simulink model "IsolatedUDP_v2"  (R2020a)
settings: Solver=FixedStepAuto  StartTime=0.0  StopTime=inf  FixedStep=0.001  RelTol=1e-3  EnableMultiTasking=on
undefined symbols (not defined in the file): daq
libraries: instrumentlib x2, dspstat3 x2, dspsigops x2, daqlib x1, quarc_library x1
settings Model: SimulationMode=accelerator  ExtModeTrigDuration=10000  Creator=pthms  LastModifiedBy=jacksonbremen
settings SolverCC: ConcurrentTasks=on  PositivePriorityOrder=on  AutoInsertRateTranBlk=on  InsertRTBMode=Never (minimum delay)
settings DataIOCC: ReturnWorkspaceOutputs=off
settings DebuggingCC: ArithmeticOperatorsInVariantConditions=warning
settings SFSimCC: SimUseLocalCustomCode=off  CustomCodeUndefinedFunction=UseInterfaceOnly
settings RTWCC: Description=QUARC Win64 Target  SystemTargetFile=quarc_win64.tlc  TemplateMakefile=quarc_default_tmf  RTWUseLocalCustomCode=off
settings STFCustomTargetCC: TargetPreCompLibLocation=C:\PROGRA~3\QUARC\lib\2018a\win64\release  TargetLangStandard=C99 (ISO)  ConcurrentExecutionCompliant=on  GRTInterface=on  SystemTargetFile=quarc_win64.tlc
settings GRTTargetCC: TargetPreCompLibLocation=C:\PROGRA~3\QUARC\lib\2018a\win64\release  ParMdlRefBuildCompliant=off  CompOptLevelCompliant=off  CombineOutputUpdateFcns=off  MatFileLogging=off  CPPClassGenCompliant=off  GRTInterface=on  UseToolchainInfoCompliant=off  ExtMode=on  ExtModeMexFile=quarc_comm

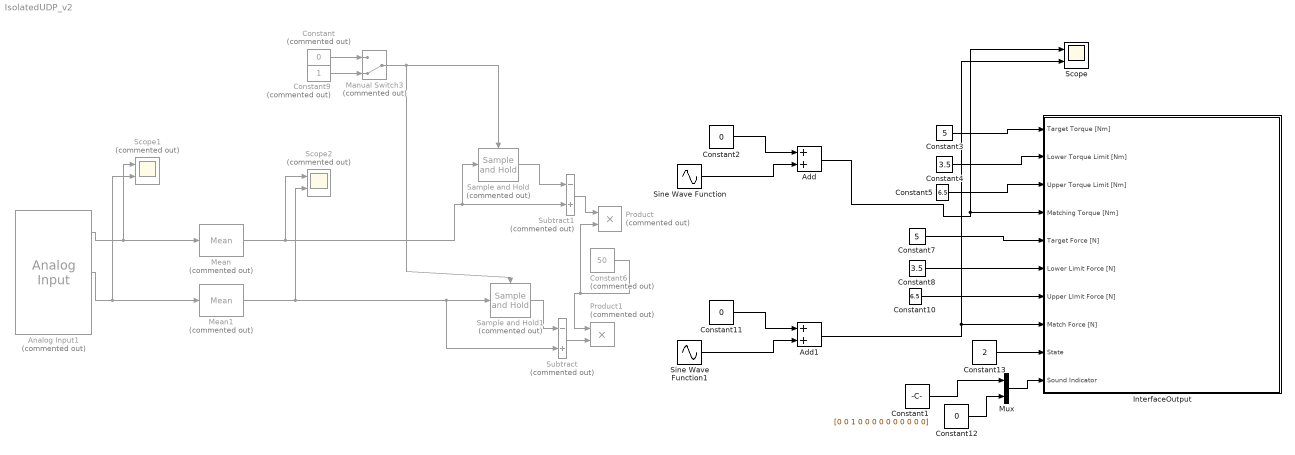
== system IsolatedUDP_v2 ==
  Add : Sum
  Add1 : Sum
  Analog Input1 : daqlib/Analog Input  Commented=on  DeviceMenu=ni Dev1 (USB-6229 (OEM))  Device=ni Dev1 (USB-6229 (OEM))  ObjConstructor=daq.createSession('ni')  NChannelsSelected=2  Channels=1$ai0$$Dev1$1$4$3$1$#1$ai1$$Dev1$1$4$3$1$#0$ai2$$Dev1$1$4$3$1$#0$ai3$$Dev1$1$4$3$1$#0$ai4$$Dev1$1$4$3$1$#0$ai5$$Dev1$1$4$3$1$#0$ai6$$Dev1$1$4$3$1$#0$ai7$$Dev1$1$4$3$1$#0$ai8$$Dev1$1$4$1$1$#0$ai9$$Dev1$1$4$1$1$#0$ai10$$Dev1$1$4$1$1$#0$ai11$$Dev1$1$4$1$1$#0$ai12$$Dev1$1$4$1$1$#0$ai13$$Dev1$1$4$1$1$#0$ai14$$Dev1$1$4$1$1$#0$ai15$$Dev1$1$4$1$1$#0$ai16$$Dev1$1$4$3$1$#0$ai17$$Dev1$1$4$3$1$#0$ai18$$Dev1$1$4$3$1$#0$ai19$$Dev1$1$4$3$1$#0$ai20$$Dev1$1$4$3$1$#0$ai21$$Dev1$1$4$3$1$#0$ai22$$Dev1$1$4$3$1$#0$ai23$$Dev1$1$4$3$1$#0$ai24$$Dev1$1$4$1$1$#0$ai25$$Dev1$1$4$1$1$#0$ai26$$Dev1$1$4$1$1$#0$ai27$$Dev1$1$4$1$1$#0$ai28$$Dev1$1$4$1$1$#0$ai29$$Dev1$1$4$1$1$#0$ai30$$Dev1$1$4$1$1$#0$ai31$$Dev1$1$4$1$1$#  NPorts=1 per channel  SampleRate=1000  ActualRate=1000  ScansPerTrigger=20  OutputTimestamp=on  AcqMode=1  NumFrameBuffer=100  OutputTriggertime=off
      settings: SourceProductBaseCode=DA
  Constant : Constant  Commented=on  Value=0
  Constant1 : Constant  Value=[0 0 1 0 0 0 0 0 0 0 0 0 0]  VectorParams1D=off  OutDataTypeStr=uint8
  Constant10 : Constant  Value=6.5  OutDataTypeStr=double
  Constant11 : Constant  Value=0  OutDataTypeStr=double
  Constant12 : Constant  Value=0  OutDataTypeStr=uint8
  Constant13 : Constant  Value=2  OutDataTypeStr=uint8
  Constant2 : Constant  Value=0  OutDataTypeStr=double
  Constant3 : Constant  Value=5  OutDataTypeStr=double
  Constant4 : Constant  Value=3.5  OutDataTypeStr=double
  Constant5 : Constant  Value=6.5  OutDataTypeStr=double
  Constant6 : Constant  Commented=on  Value=50
  Constant7 : Constant  Value=5  OutDataTypeStr=double
  Constant8 : Constant  Value=3.5  OutDataTypeStr=double
  Constant9 : Constant  Commented=on
  InterfaceOutput : Subsystem
      mask Display: color('blue');disp('Interface Output Stream \nUDP');
  Manual Switch3 : ManualSwitch  Commented=on  CurrentSetting=0
  Mean : dspstat3/Mean  Commented=on  run=off  InputProcessing=Columns as channels (frame based)  reset_popup=None  directionMode=Each column  dimension=1  roiEnable=off  roiType=Rectangles  roiPortion=Entire ROI  roiOutput=Individual statistics for each ROI  roiFlag=off  roundingMode=Floor  overflowMode=off  outputDataTypeStr=Inherit: Same as accumulator  outputMin=[]  outputMax=[]  outputLastDataTypeStr=Inherit: Same as accumulator
  Mean1 : dspstat3/Mean  Commented=on  run=off  InputProcessing=Columns as channels (frame based)  reset_popup=None  directionMode=Each column  dimension=1  roiEnable=off  roiType=Rectangles  roiPortion=Entire ROI  roiOutput=Individual statistics for each ROI  roiFlag=off  roundingMode=Floor  overflowMode=off  outputDataTypeStr=Inherit: Same as accumulator  outputMin=[]  outputMax=[]  outputLastDataTypeStr=Inherit: Same as accumulator
  Mux : Mux  Inputs=2
  Product : Product  Commented=on
  Product1 : Product  Commented=on
  Sample and Hold : dspsigops/Sample and Hold  Commented=on  trig=Either edge  initCond=0  latchinput=off
  Sample and Hold1 : dspsigops/Sample and Hold  Commented=on  trig=Either edge  initCond=0  latchinput=off
  Scope : Scope  NumInputPorts=2
  Scope1 : Scope  Commented=on  NumInputPorts=2
  Scope2 : Scope  Commented=on  NumInputPorts=2
  Sine Wave Function : Sin  Amplitude=7  Frequency=0.5  SampleTime=0
  Sine Wave Function1 : Sin  Amplitude=5  Bias=5  Frequency=0.5  Phase=pi/3  SampleTime=0
  Subtract : Sum  Commented=on  Inputs=-+
  Subtract1 : Sum  Commented=on  Inputs=-+
  wires:
  Constant3/1 -> InterfaceOutput/1(Target Torque [Nm])
  Constant4/1 -> InterfaceOutput/2(Lower Torque Limit [Nm])
  Constant5/1 -> InterfaceOutput/3(Upper Torque Limit [Nm])
  Constant2/1 -> Add/1
  Sine Wave Function/1 -> Add/2
  Constant6/1 -> Product1/1, Product/2
  Constant7/1 -> InterfaceOutput/5(Target Force [N])
  Constant8/1 -> InterfaceOutput/6(Lower Limit Force [N])
  Constant10/1 -> InterfaceOutput/7(Upper LImit Force [N])
  Subtract/1 -> Product1/2
  Add/1 -> Scope/1, InterfaceOutput/4(Matching Torque [Nm])
  Add1/1 -> Scope/2, InterfaceOutput/8(Match Force [N])
  Subtract1/1 -> Product/1
  Mean1/1 -> Scope2/2, Subtract/2, Sample and Hold1/1
  Mean/1 -> Scope2/1, Sample and Hold/1, Subtract1/2
  Analog Input1/1 -> Mean/1, Scope1/1
  Analog Input1/2 -> Mean1/1, Scope1/2
  Constant/1 -> Manual Switch3/1
  Manual Switch3/1 -> Sample and Hold1/Trigger, Sample and Hold/Trigger
  Constant9/1 -> Manual Switch3/2
  Sample and Hold/1 -> Subtract1/1
  Sample and Hold1/1 -> Subtract/1
  Sine Wave Function1/1 -> Add1/2
  Constant11/1 -> Add1/1
  Constant1/1 -> Mux/1
  Mux/1 -> InterfaceOutput/10(Sound Indicator)
  Constant12/1 -> Mux/2
  Constant13/1 -> InterfaceOutput/9(State)

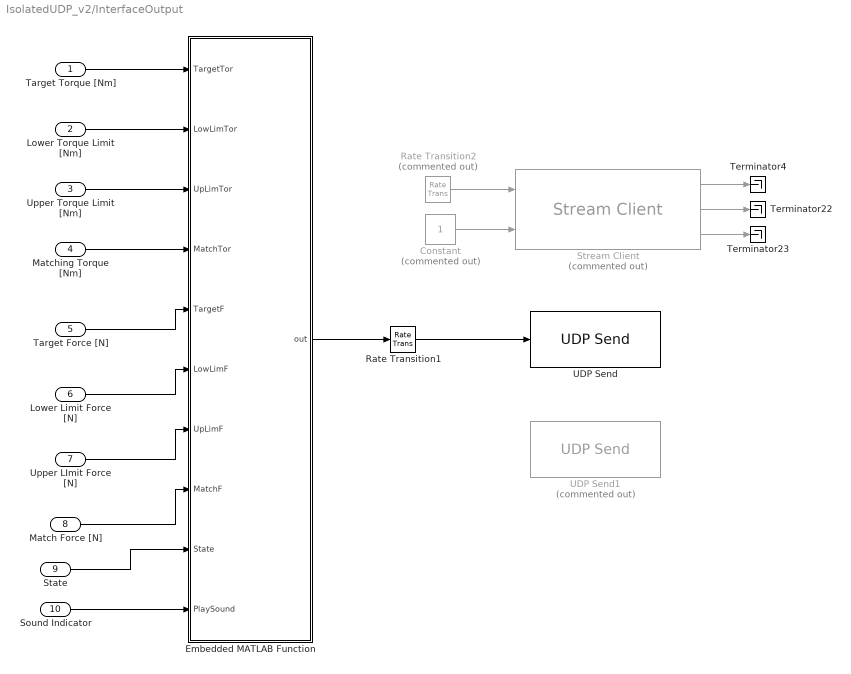
== system IsolatedUDP_v2/InterfaceOutput ==
  Target Torque [Nm] : Inport
  Lower Torque Limit [Nm] : Inport  Port=2
  Upper Torque Limit [Nm] : Inport  Port=3
  Matching Torque [Nm] : Inport  Port=4
  Target Force [N] : Inport  Port=5
  Lower Limit Force [N] : Inport  Port=6
  Upper LImit Force [N] : Inport  Port=7
  Match Force [N] : Inport  Port=8
  State : Inport  Port=9
  Sound Indicator : Inport  Port=10
  Constant : Constant  Commented=on
  Embedded MATLAB Function : MATLAB Function  TreatAsAtomicUnit=on
  Rate Transition1 : RateTransition  Deterministic=off  OutPortSampleTime=0.01
  Rate Transition2 : RateTransition  Commented=on  OutPortSampleTime=0.01
  Stream Client : quarc_library/Communications/Basic/Stream Client  Commented=on  uri_source=Specify via dialog (do not evaluate)  uri=udp://192.168.0.103:25000  apply_uri_to_all_configs=on  send_buffer_size=1460  receive_buffer_size=1460  byte_order=little endian (Intel - LSB first)  optimization=Minimum latency  send_options=Send all data  receive_options=Do not receive data  default_value=[0]  sample_time=0.01  active=on  implementation=Use non-blocking I/O  send_fifo_size=1000  receive_fifo_size=1000  send_priority=0  receive_priority=0  send_dimensions=off  receive_dimensions=off  max_dimensions=-1  data_type=Inherited via back propagation  type_expr=BusObject
      settings: AttributesFormatString="\"udp://192.168.0.103:25000\""
  Terminator22 : Terminator
  Terminator23 : Terminator
  Terminator4 : Terminator
  UDP Send : instrumentlib/UDP Send  Host=165.124.9.111  Port=5005  LocalPort=-1  EnablePortSharing=off  ByteOrder=LittleEndian  OutputDatagramPacketSize=1460  EnableBlockingMode=off  LocalAddress=0.0.0.0
  UDP Send1 : instrumentlib/UDP Send  Commented=on  Host=localhost  Port=5005  LocalPort=-1  EnablePortSharing=off  ByteOrder=LittleEndian  OutputDatagramPacketSize=1460  EnableBlockingMode=off  LocalAddress=0.0.0.0
  wires:
  Constant/1 -> Stream Client/2
  Stream Client/1 -> Terminator4/1
  Stream Client/2 -> Terminator22/1
  Stream Client/3 -> Terminator23/1
  Target Torque [Nm]/1 -> Embedded MATLAB Function/1(TargetTor)
  Lower Torque Limit [Nm]/1 -> Embedded MATLAB Function/2(LowLimTor)
  Upper Torque Limit [Nm]/1 -> Embedded MATLAB Function/3(UpLimTor)
  Matching Torque [Nm]/1 -> Embedded MATLAB Function/4(MatchTor)
  Sound Indicator/1 -> Embedded MATLAB Function/10(PlaySound)
  Match Force [N]/1 -> Embedded MATLAB Function/8(MatchF)
  Upper LImit Force [N]/1 -> Embedded MATLAB Function/7(UpLimF)
  Lower Limit Force [N]/1 -> Embedded MATLAB Function/6(LowLimF)
  Target Force [N]/1 -> Embedded MATLAB Function/5(TargetF)
  Embedded MATLAB Function/1(out) -> Rate Transition1/1
  Rate Transition1/1 -> UDP Send/1
  Rate Transition2/1 -> Stream Client/1
  State/1 -> Embedded MATLAB Function/9(State)

== matlab function IsolatedUDP_v2/InterfaceOutput/Embedded MATLAB Function ==
  data: TargetTor input; LowLimTor input; UpLimTor input; MatchTor input; TargetF input; LowLimF input; UpLimF input; MatchF input; State input; PlaySound input; out output uint8
%function out = fcn(TargetTor,LowLimTor,UpLimTor,MatchTor,PlaySound)

function out = fcn(TargetTor,LowLimTor,UpLimTor,MatchTor,TargetF, LowLimF, UpLimF, MatchF, State, PlaySound)

%     out = uint8(zeros(4*8+14,1));
% 
%     out(1:8)    = uint8(typecast(double(TargetTor),'uint8'));
%     out(9:16)   = uint8(typecast(double(LowLimTor),'uint8'));
%     out(17:24)  = uint8(typecast(double(UpLimTor),'uint8'));
%     out(25:32)  = uint8(typecast(double(MatchTor),'uint8'));
% 
%     out(33:46)  = uint8(typecast(uint8(PlaySound(1:14)),'uint8'));
%     
    out = uint8(zeros(8*9+14,1));

    out(1:8)    = uint8(typecast(double(TargetTor),'uint8'));
    out(9:16)   = uint8(typecast(double(LowLimTor),'uint8'));
    out(17:24)  = uint8(typecast(double(UpLimTor),'uint8'));
    out(25:32)  = uint8(typecast(double(MatchTor),'uint8'));
    
    out(33:40)    = uint8(typecast(double(TargetF),'uint8'));
    out(41:48)   = uint8(typecast(double(LowLimF),'uint8'));
    out(49:56)  = uint8(typecast(double(UpLimF),'uint8'));
    out(57:64)  = uint8(typecast(double(MatchF),'uint8'));
    out(65:72) = uint8(typecast(double(State),'uint8'));
    
    % PlaySoound will not be predefined in the real thing
%     PlaySound = zeros(1, 14);
%     PlaySound(4) = 1;
    out(73:86)  = uint8(typecast(uint8(PlaySound(1:14)),'uint8'));
%     
end
